simulink model "ackerman_ROS_neural_controller"  (R2023b)
settings: Solver=FixedStepDiscrete  StartTime=0.0  StopTime=20  FixedStep=0.1  RelTol=1e-3
undefined symbols (not defined in the file or in its folder): Angular, Linear
libraries: neural x61, robotlib x15, robotcorelib x1
(part 2 of 3)

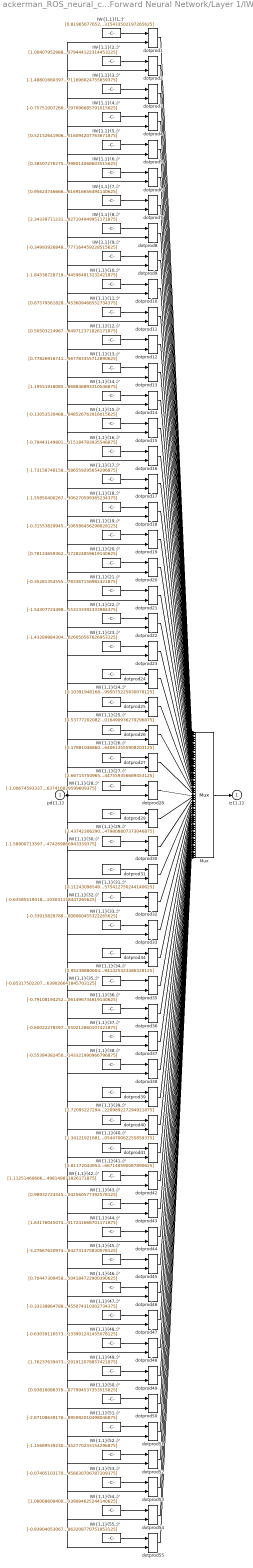
== system ackerman_ROS_neural_controller/Controlador/Feed-Forward Neural Network/Layer 1/IW{1,1} ==
  "pd{1,1}" : Inport  PortDimensions=7
      mask Display: e = 0.06;c1 = [120 230 180]/255;c2 = ([120 230 180]+0)/(256+128);c3 = ([120 230 180]+128)/(256+128);patch([0 1 1 0],[0 0 1 1],c1);patch([0 1 1 1-e 1-e 0+e],[0 0 1 1-e 0+e 0+e],c2);patch([0 0 1 1-e 0+e 0+e],[0 1 1 1-e 1-e 0+e],c3);plot([0 1 1 0 0],[0 0 1 1 0]);
  "IW{1,1}(1,:)'" : Constant  Value=[0.8196567765200553079552037161192856729030609130859375;-1.926081750277442328211918720626272261142730712890625;0.00937690139589171522960242555200238712131977081298828125;-0.99967118914263497497785238010692410171031951904296875;0.88527747342578033684645788525813259184360504150390625;-0.016050046443263653317412575916023342870175838470458984375;2.516567789495900431262498386786319315433502197265625]
      mask Display: e = 0.06;c1 = [120 150 230]/255;c2 = ([120 150 230]+0)/383;c3 = ([120 150 230]+128)/383;patch([0 1 1 0],[0 0 1 1],c1);patch([0 1 1 1-e 1-e 0+e],[0 0 1 1-e 0+e 0+e],c2);patch([0 0 1 1-e 0+e 0+e],[0 1 1 1-e 1-e 0+e],c3);plot([0 1 1 0 0],[0 0 1 1 0]);disp('Weights');
  "IW{1,1}(10,:)'" : Constant  Value=[-1.8453872871921481735313363969908095896244049072265625;1.7100070055517571088188333305879496037960052490234375;-1.2349725100067565630723720460082404315471649169921875;-0.3362332664637464052503901257296092808246612548828125;-1.5013049550553019262366660768748261034488677978515625;0.8324461871242399002568390642409212887287139892578125;-0.88812634608944385217199624094064347445964813232421875]
      mask Display: e = 0.06;c1 = [120 150 230]/255;c2 = ([120 150 230]+0)/383;c3 = ([120 150 230]+128)/383;patch([0 1 1 0],[0 0 1 1],c1);patch([0 1 1 1-e 1-e 0+e],[0 0 1 1-e 0+e 0+e],c2);patch([0 0 1 1-e 0+e 0+e],[0 1 1 1-e 1-e 0+e],c3);plot([0 1 1 0 0],[0 0 1 1 0]);disp('Weights');
  "IW{1,1}(11,:)'" : Constant  Value=[0.87579561828426777392309077185927890241146087646484375;-2.18084780642070175105118323699571192264556884765625;1.2546608949978901303978773285052739083766937255859375;-0.09026831162019467724721977219815016724169254302978515625;-0.07461867636167125727997273543223855085670948028564453125;-0.00755235780173457715847007420961745083332061767578125;0.464016361247922670685284174396656453609466552734375]
      mask Display: e = 0.06;c1 = [120 150 230]/255;c2 = ([120 150 230]+0)/383;c3 = ([120 150 230]+128)/383;patch([0 1 1 0],[0 0 1 1],c1);patch([0 1 1 1-e 1-e 0+e],[0 0 1 1-e 0+e 0+e],c2);patch([0 0 1 1-e 0+e 0+e],[0 1 1 1-e 1-e 0+e],c3);plot([0 1 1 0 0],[0 0 1 1 0]);disp('Weights');
  "IW{1,1}(12,:)'" : Constant  Value=[0.5050321496787890662716336009907536208629608154296875;0.328844036297810060620605554504436440765857696533203125;1.77708828566390497627480726805515587329864501953125;-1.3961094208468234345588143696659244596958160400390625;0.28492086151952722428148945255088619887828826904296875;1.5220770934261285134425634169019758701324462890625;-0.064043810457246663769836914070765487849712371826171875]
      mask Display: e = 0.06;c1 = [120 150 230]/255;c2 = ([120 150 230]+0)/383;c3 = ([120 150 230]+128)/383;patch([0 1 1 0],[0 0 1 1],c1);patch([0 1 1 1-e 1-e 0+e],[0 0 1 1-e 0+e 0+e],c2);patch([0 0 1 1-e 0+e 0+e],[0 1 1 1-e 1-e 0+e],c3);plot([0 1 1 0 0],[0 0 1 1 0]);disp('Weights');
  "IW{1,1}(13,:)'" : Constant  Value=[0.77826916741648866082670110699837096035480499267578125;-0.6526054454813519090095041974564082920551300048828125;1.551566772193030185889028871315531432628631591796875;1.1956969864732924779815448346198536455631256103515625;-1.4944987700257410523363432730548083782196044921875;1.1012912516788346817264709898154251277446746826171875;-0.1254181577627761223769908838221454061567783355712890625]
      mask Display: e = 0.06;c1 = [120 150 230]/255;c2 = ([120 150 230]+0)/383;c3 = ([120 150 230]+128)/383;patch([0 1 1 0],[0 0 1 1],c1);patch([0 1 1 1-e 1-e 0+e],[0 0 1 1-e 0+e 0+e],c2);patch([0 0 1 1-e 0+e 0+e],[0 1 1 1-e 1-e 0+e],c3);plot([0 1 1 0 0],[0 0 1 1 0]);disp('Weights');
  "IW{1,1}(14,:)'" : Constant  Value=[1.195519180856158936165911654825322329998016357421875;1.2214638332623959371403543627820909023284912109375;1.6603997501206200215762009975151158869266510009765625;2.570219412985425666562377955415286123752593994140625;-0.81621421998230847538735588386771269142627716064453125;0.106969592196890561641708927709260024130344390869140625;-0.2002481022235455820901250945098581723868846893310546875]
      mask Display: e = 0.06;c1 = [120 150 230]/255;c2 = ([120 150 230]+0)/383;c3 = ([120 150 230]+128)/383;patch([0 1 1 0],[0 0 1 1],c1);patch([0 1 1 1-e 1-e 0+e],[0 0 1 1-e 0+e 0+e],c2);patch([0 0 1 1-e 0+e 0+e],[0 1 1 1-e 1-e 0+e],c3);plot([0 1 1 0 0],[0 0 1 1 0]);disp('Weights');
  "IW{1,1}(15,:)'" : Constant  Value=[-0.1305353046822148310734945653166505508124828338623046875;0.42887859104116843322884733424871228635311126708984375;-0.1528195850874631833704597738687880337238311767578125;-0.44812624061969741351418861086131073534488677978515625;2.323367873082375911764074771781452000141143798828125;0.09038873200569443044916084772921749390661716461181640625;1.265699700169220509593515089363791048526763916015625]
      mask Display: e = 0.06;c1 = [120 150 230]/255;c2 = ([120 150 230]+0)/383;c3 = ([120 150 230]+128)/383;patch([0 1 1 0],[0 0 1 1],c1);patch([0 1 1 1-e 1-e 0+e],[0 0 1 1-e 0+e 0+e],c2);patch([0 0 1 1-e 0+e 0+e],[0 1 1 1-e 1-e 0+e],c3);plot([0 1 1 0 0],[0 0 1 1 0]);disp('Weights');
  "IW{1,1}(16,:)'" : Constant  Value=[-0.79443149801045287450307341714506037533283233642578125;-1.2581818433612481644701119876117445528507232666015625;0.403920568372703014947688870961428619921207427978515625;-0.9387576041271177285096882769721560180187225341796875;-1.0760361386877399514361286492203362286090850830078125;0.02723946620754004455111640936593175865709781646728515625;2.420834616643684267245362207177095115184783935546875]
      mask Display: e = 0.06;c1 = [120 150 230]/255;c2 = ([120 150 230]+0)/383;c3 = ([120 150 230]+128)/383;patch([0 1 1 0],[0 0 1 1],c1);patch([0 1 1 1-e 1-e 0+e],[0 0 1 1-e 0+e 0+e],c2);patch([0 0 1 1-e 0+e 0+e],[0 1 1 1-e 1-e 0+e],c3);plot([0 1 1 0 0],[0 0 1 1 0]);disp('Weights');
  "IW{1,1}(17,:)'" : Constant  Value=[-1.731587481587970156482469974434934556484222412109375;-1.2350643156762668439796470920555293560028076171875;-0.50287132855106786433196930374833755195140838623046875;-0.52530204840375471775359983439557254314422607421875;1.43947154865100213072537371772341430187225341796875;0.04561385884697267967258227372440160252153873443603515625;0.50957825059342443108079123703646473586559295654296875]
      mask Display: e = 0.06;c1 = [120 150 230]/255;c2 = ([120 150 230]+0)/383;c3 = ([120 150 230]+128)/383;patch([0 1 1 0],[0 0 1 1],c1);patch([0 1 1 1-e 1-e 0+e],[0 0 1 1-e 0+e 0+e],c2);patch([0 0 1 1-e 0+e 0+e],[0 1 1 1-e 1-e 0+e],c3);plot([0 1 1 0 0],[0 0 1 1 0]);disp('Weights');
  "IW{1,1}(18,:)'" : Constant  Value=[-1.5585040026759988673887846744037233293056488037109375;0.109992370714509901663546997951925732195377349853515625;0.82737968051371080235867339069955050945281982421875;1.900815407616306629279279150068759918212890625;0.1491678806411325941549961271448410116136074066162109375;-1.205691924855796681725905727944336831569671630859375;0.060510711771919911683426107629202306270599365234375]
      mask Display: e = 0.06;c1 = [120 150 230]/255;c2 = ([120 150 230]+0)/383;c3 = ([120 150 230]+128)/383;patch([0 1 1 0],[0 0 1 1],c1);patch([0 1 1 1-e 1-e 0+e],[0 0 1 1-e 0+e 0+e],c2);patch([0 0 1 1-e 0+e 0+e],[0 1 1 1-e 1-e 0+e],c3);plot([0 1 1 0 0],[0 0 1 1 0]);disp('Weights');
  "IW{1,1}(19,:)'" : Constant  Value=[-0.315538299455872917054222170918365009129047393798828125;0.259542684982053406539392881313688121736049652099609375;-1.2126404532456895868364199486677534878253936767578125;-5.8374282487121842422084228019230067729949951171875;2.580560676999312352819515581359155476093292236328125;0.54278960426659172977537082260823808610439300537109375;-0.8672580816556649807580470223911106586456298828125]
      mask Display: e = 0.06;c1 = [120 150 230]/255;c2 = ([120 150 230]+0)/383;c3 = ([120 150 230]+128)/383;patch([0 1 1 0],[0 0 1 1],c1);patch([0 1 1 1-e 1-e 0+e],[0 0 1 1-e 0+e 0+e],c2);patch([0 0 1 1-e 0+e 0+e],[0 1 1 1-e 1-e 0+e],c3);plot([0 1 1 0 0],[0 0 1 1 0]);disp('Weights');
  "IW{1,1}(2,:)'" : Constant  Value=[1.00407952988688276008133470895700156688690185546875;1.752935551171999950526014799834229052066802978515625;-1.414218430030616868720017009763978421688079833984375;-0.25046873033662586660597071386291645467281341552734375;-1.9154355127652473722577042281045578420162200927734375;0.1438730267330297907246716704321443103253841400146484375;-0.310184078325510814710952445238945074379444122314453125]
      mask Display: e = 0.06;c1 = [120 150 230]/255;c2 = ([120 150 230]+0)/383;c3 = ([120 150 230]+128)/383;patch([0 1 1 0],[0 0 1 1],c1);patch([0 1 1 1-e 1-e 0+e],[0 0 1 1-e 0+e 0+e],c2);patch([0 0 1 1-e 0+e 0+e],[0 1 1 1-e 1-e 0+e],c3);plot([0 1 1 0 0],[0 0 1 1 0]);disp('Weights');
  "IW{1,1}(20,:)'" : Constant  Value=[0.78124659362565151976554034263244830071926116943359375;0.289651182914616500685411892845877446234226226806640625;-1.350122749788877474230730513227172195911407470703125;-1.5462269165205555498943112979759462177753448486328125;0.32235172181962690185486053451313637197017669677734375;-0.5104310959630049548962915650918148458003997802734375;1.810732280847093367270872477092780172824859619140625]
      mask Display: e = 0.06;c1 = [120 150 230]/255;c2 = ([120 150 230]+0)/383;c3 = ([120 150 230]+128)/383;patch([0 1 1 0],[0 0 1 1],c1);patch([0 1 1 1-e 1-e 0+e],[0 0 1 1-e 0+e 0+e],c2);patch([0 0 1 1-e 0+e 0+e],[0 1 1 1-e 1-e 0+e],c3);plot([0 1 1 0 0],[0 0 1 1 0]);disp('Weights');
  "IW{1,1}(21,:)'" : Constant  Value=[-0.35281354555303534592525238622329197824001312255859375;0.1032751127231832100061836854365537874400615692138671875;0.169498037490068476085269821851397864520549774169921875;-1.163129210222102916105768599663861095905303955078125;-1.516689324515800851855829023406840860843658447265625;-1.50230615007458201404233477660454809665679931640625;0.9213137951345735654484769838745705783367156982421875]
      mask Display: e = 0.06;c1 = [120 150 230]/255;c2 = ([120 150 230]+0)/383;c3 = ([120 150 230]+128)/383;patch([0 1 1 0],[0 0 1 1],c1);patch([0 1 1 1-e 1-e 0+e],[0 0 1 1-e 0+e 0+e],c2);patch([0 0 1 1-e 0+e 0+e],[0 1 1 1-e 1-e 0+e],c3);plot([0 1 1 0 0],[0 0 1 1 0]);disp('Weights');
  "IW{1,1}(22,:)'" : Constant  Value=[-1.543077244984001783478788638603873550891876220703125;1.840093239849561967957924935035407543182373046875;-1.5256171026490890074711614943225868046283721923828125;-0.51244468639139062471343777360743843019008636474609375;0.637896693551966986746037946431897580623626708984375;0.8300709977513041071262023251620121300220489501953125;-1.3458241602968799011108558261184953153133392333984375]
      mask Display: e = 0.06;c1 = [120 150 230]/255;c2 = ([120 150 230]+0)/383;c3 = ([120 150 230]+128)/383;patch([0 1 1 0],[0 0 1 1],c1);patch([0 1 1 1-e 1-e 0+e],[0 0 1 1-e 0+e 0+e],c2);patch([0 0 1 1-e 0+e 0+e],[0 1 1 1-e 1-e 0+e],c3);plot([0 1 1 0 0],[0 0 1 1 0]);disp('Weights');
  "IW{1,1}(23,:)'" : Constant  Value=[-1.43289884304300851880498157697729766368865966796875;1.9791366659345455136786995353759266436100006103515625;0.481076891871465461836265831152559258043766021728515625;-1.2587924341996383770236889176885597407817840576171875;0.2231337452412995581152443946848507039248943328857421875;1.2838954097952697264162225110339932143688201904296875;0.97161406138600459048149105001357384026050567626953125]
      mask Display: e = 0.06;c1 = [120 150 230]/255;c2 = ([120 150 230]+0)/383;c3 = ([120 150 230]+128)/383;patch([0 1 1 0],[0 0 1 1],c1);patch([0 1 1 1-e 1-e 0+e],[0 0 1 1-e 0+e 0+e],c2);patch([0 0 1 1-e 0+e 0+e],[0 1 1 1-e 1-e 0+e],c3);plot([0 1 1 0 0],[0 0 1 1 0]);disp('Weights');
  "IW{1,1}(24,:)'" : Constant  Value=[0.1039194816821370215276232329415506683290004730224609375;-2.24536042172727778876151205622591078281402587890625;0.94414930025091425846994752646423876285552978515625;-0.472618055494270716820892630494199693202972412109375;0.7174481316047778278743862756527960300445556640625;2.271186922768583027476552160806022584438323974609375;2.795885435963406440151857168530113995075225830078125]
      mask Display: e = 0.06;c1 = [120 150 230]/255;c2 = ([120 150 230]+0)/383;c3 = ([120 150 230]+128)/383;patch([0 1 1 0],[0 0 1 1],c1);patch([0 1 1 1-e 1-e 0+e],[0 0 1 1-e 0+e 0+e],c2);patch([0 0 1 1-e 0+e 0+e],[0 1 1 1-e 1-e 0+e],c3);plot([0 1 1 0 0],[0 0 1 1 0]);disp('Weights');
  "IW{1,1}(25,:)'" : Constant  Value=[0.53777202082343311673184871324338018894195556640625;0.52823704471663857074048564754775725305080413818359375;-0.59883371214820979577808657268178649246692657470703125;0.12258232964106541285076446001767180860042572021484375;0.5166091212520906861271896559628657996654510498046875;-0.13458293841771162835385666767251677811145782470703125;0.8974266232529461984057661538827233016490936279296875]
      mask Display: e = 0.06;c1 = [120 150 230]/255;c2 = ([120 150 230]+0)/383;c3 = ([120 150 230]+128)/383;patch([0 1 1 0],[0 0 1 1],c1);patch([0 1 1 1-e 1-e 0+e],[0 0 1 1-e 0+e 0+e],c2);patch([0 0 1 1-e 0+e 0+e],[0 1 1 1-e 1-e 0+e],c3);plot([0 1 1 0 0],[0 0 1 1 0]);disp('Weights');
  "IW{1,1}(26,:)'" : Constant  Value=[0.1788104686056406766869741886694100685417652130126953125;0.330006955410862834465746118439710699021816253662109375;-1.1674892308520219419420982376323081552982330322265625;-2.918953004432601527895485560293309390544891357421875;1.1324442299923582755383222320233471691608428955078125;0.7442867829941091084577919900766573846340179443359375;-0.361699594847931404917318332081777043640613555908203125]
      mask Display: e = 0.06;c1 = [120 150 230]/255;c2 = ([120 150 230]+0)/383;c3 = ([120 150 230]+128)/383;patch([0 1 1 0],[0 0 1 1],c1);patch([0 1 1 1-e 1-e 0+e],[0 0 1 1-e 0+e 0+e],c2);patch([0 0 1 1-e 0+e 0+e],[0 1 1 1-e 1-e 0+e],c3);plot([0 1 1 0 0],[0 0 1 1 0]);disp('Weights');
  "IW{1,1}(27,:)'" : Constant  Value=[2.66715750965894660140520500135608017444610595703125;-2.27722146233000888315700649400241672992706298828125;0.71597217798577694747308441947097890079021453857421875;-1.6139328980116334211203366066911257803440093994140625;1.9382503882814037243775828756042756140232086181640625;-0.2017845621484758711350337989642866887152194976806640625;0.08781462402644509002147543696992215700447559356689453125]
      mask Display: e = 0.06;c1 = [120 150 230]/255;c2 = ([120 150 230]+0)/383;c3 = ([120 150 230]+128)/383;patch([0 1 1 0],[0 0 1 1],c1);patch([0 1 1 1-e 1-e 0+e],[0 0 1 1-e 0+e 0+e],c2);patch([0 0 1 1-e 0+e 0+e],[0 1 1 1-e 1-e 0+e],c3);plot([0 1 1 0 0],[0 0 1 1 0]);disp('Weights');
  "IW{1,1}(28,:)'" : Constant  Value=[-1.006745933372045431752894728560931980609893798828125;-2.0608963324433648978128985618241131305694580078125;0.043165708065044106067631446421728469431400299072265625;0.719486909065246482697375540737994015216827392578125;-0.1733343365394100776821773024494177661836147308349609375;-0.2415300122648019465199098476659855805337429046630859375;-1.1204520286378620852474341518245637416839599609375]
      mask Display: e = 0.06;c1 = [120 150 230]/255;c2 = ([120 150 230]+0)/383;c3 = ([120 150 230]+128)/383;patch([0 1 1 0],[0 0 1 1],c1);patch([0 1 1 1-e 1-e 0+e],[0 0 1 1-e 0+e 0+e],c2);patch([0 0 1 1-e 0+e 0+e],[0 1 1 1-e 1-e 0+e],c3);plot([0 1 1 0 0],[0 0 1 1 0]);disp('Weights');
  "IW{1,1}(29,:)'" : Constant  Value=[2.437423062906741488831130482139997184276580810546875;-2.356093352610267199764848555787466466426849365234375;-1.750998763544374892120458753197453916072845458984375;0.1934240615399113460970426103813224472105503082275390625;-0.11899669455935434070337208822820684872567653656005859375;1.12619821571909550783630038495175540447235107421875;3.56357954247615094089951526257209479808807373046875]
      mask Display: e = 0.06;c1 = [120 150 230]/255;c2 = ([120 150 230]+0)/383;c3 = ([120 150 230]+128)/383;patch([0 1 1 0],[0 0 1 1],c1);patch([0 1 1 1-e 1-e 0+e],[0 0 1 1-e 0+e 0+e],c2);patch([0 0 1 1-e 0+e 0+e],[0 1 1 1-e 1-e 0+e],c3);plot([0 1 1 0 0],[0 0 1 1 0]);disp('Weights');
  "IW{1,1}(3,:)'" : Constant  Value=[-1.4880166039728168758671245086588896811008453369140625;0.245406596910593799432120931669487617909908294677734375;-0.651966682995968493941063570673577487468719482421875;-0.2076135471464277681974408551468513906002044677734375;-0.9089205659120456193278414502856321632862091064453125;1.1562892851109205505366617217077873647212982177734375;-0.6555946798450447143835617680451832711696624755859375]
      mask Display: e = 0.06;c1 = [120 150 230]/255;c2 = ([120 150 230]+0)/383;c3 = ([120 150 230]+128)/383;patch([0 1 1 0],[0 0 1 1],c1);patch([0 1 1 1-e 1-e 0+e],[0 0 1 1-e 0+e 0+e],c2);patch([0 0 1 1-e 0+e 0+e],[0 1 1 1-e 1-e 0+e],c3);plot([0 1 1 0 0],[0 0 1 1 0]);disp('Weights');
  "IW{1,1}(30,:)'" : Constant  Value=[-1.589007135976476359218167999642901122570037841796875;-1.31141949337409879916549471090547740459442138671875;-1.0226840662479588228706006702850572764873504638671875;1.7847567115081093280792856603511609137058258056640625;-0.9266439972251323542451473258552141487598419189453125;-0.00035821150614343856555255030116313719190657138824462890625;1.7299014906363507915187938124290667474269866943359375]
      mask Display: e = 0.06;c1 = [120 150 230]/255;c2 = ([120 150 230]+0)/383;c3 = ([120 150 230]+128)/383;patch([0 1 1 0],[0 0 1 1],c1);patch([0 1 1 1-e 1-e 0+e],[0 0 1 1-e 0+e 0+e],c2);patch([0 0 1 1-e 0+e 0+e],[0 1 1 1-e 1-e 0+e],c3);plot([0 1 1 0 0],[0 0 1 1 0]);disp('Weights');
  "IW{1,1}(31,:)'" : Constant  Value=[0.1124309654881923414837530117438291199505329132080078125;0.029087691018045168378503007033941685222089290618896484375;-1.055713623776400655884799562045373022556304931640625;0.93835294125979340496002123472862876951694488525390625;1.4852531373823329996497477623051963746547698974609375;-0.388212588822750614969692151134950108826160430908203125;-1.2185456909971110750490197460749186575412750244140625]
      mask Display: e = 0.06;c1 = [120 150 230]/255;c2 = ([120 150 230]+0)/383;c3 = ([120 150 230]+128)/383;patch([0 1 1 0],[0 0 1 1],c1);patch([0 1 1 1-e 1-e 0+e],[0 0 1 1-e 0+e 0+e],c2);patch([0 0 1 1-e 0+e 0+e],[0 1 1 1-e 1-e 0+e],c3);plot([0 1 1 0 0],[0 0 1 1 0]);disp('Weights');
  "IW{1,1}(32,:)'" : Constant  Value=[-0.63585519418358427135018473563832230865955352783203125;-1.5254086535969004767565593283507041633129119873046875;0.3019815538911905239416455515311099588871002197265625;0.5804630405005115623140454772510565817356109619140625;-1.937194029410040929661818154272623360157012939453125;-0.470855409083529574676418860690318979322910308837890625;-1.2814806828813607442185684703872539103031158447265625]
      mask Display: e = 0.06;c1 = [120 150 230]/255;c2 = ([120 150 230]+0)/383;c3 = ([120 150 230]+128)/383;patch([0 1 1 0],[0 0 1 1],c1);patch([0 1 1 1-e 1-e 0+e],[0 0 1 1-e 0+e 0+e],c2);patch([0 0 1 1-e 0+e 0+e],[0 1 1 1-e 1-e 0+e],c3);plot([0 1 1 0 0],[0 0 1 1 0]);disp('Weights');
  "IW{1,1}(33,:)'" : Constant  Value=[-0.33915828788690050021870092678000219166278839111328125;0.1789708238793852601578038274965365417301654815673828125;0.970370936337600742405129494727589190006256103515625;3.0714089604893803908680638414807617664337158203125;-1.5686418166151068209757113436353392899036407470703125;0.658094509689622686465781953302212059497833251953125;-1.5427494403949657542085560635314323008060455322265625]
      mask Display: e = 0.06;c1 = [120 150 230]/255;c2 = ([120 150 230]+0)/383;c3 = ([120 150 230]+128)/383;patch([0 1 1 0],[0 0 1 1],c1);patch([0 1 1 1-e 1-e 0+e],[0 0 1 1-e 0+e 0+e],c2);patch([0 0 1 1-e 0+e 0+e],[0 1 1 1-e 1-e 0+e],c3);plot([0 1 1 0 0],[0 0 1 1 0]);disp('Weights');
  "IW{1,1}(34,:)'" : Constant  Value=[0.95238880604200115698176887235604226589202880859375;-0.24816195974321664241557527930126525461673736572265625;0.322253882548174719335776217121747322380542755126953125;-1.99655520246268025630342890508472919464111328125;-1.0472174516072503269725757490959949791431427001953125;0.163076430626699797610257292035385034978389739990234375;0.66808023651050973956699863265384919941425323486328125]
      mask Display: e = 0.06;c1 = [120 150 230]/255;c2 = ([120 150 230]+0)/383;c3 = ([120 150 230]+128)/383;patch([0 1 1 0],[0 0 1 1],c1);patch([0 1 1 1-e 1-e 0+e],[0 0 1 1-e 0+e 0+e],c2);patch([0 0 1 1-e 0+e 0+e],[0 1 1 1-e 1-e 0+e],c3);plot([0 1 1 0 0],[0 0 1 1 0]);disp('Weights');
  "IW{1,1}(35,:)'" : Constant  Value=[-0.85317502207466178187900140983401797711849212646484375;-1.4926232868599556002919825914432294666767120361328125;-1.661914641538658532482486407388933002948760986328125;1.0289793115468095496822797940694727003574371337890625;-1.1862452665797944550973852528841234743595123291015625;0.75256474756981639462338762314175255596637725830078125;1.4295861162861112081401415707659907639026641845703125]
      mask Display: e = 0.06;c1 = [120 150 230]/255;c2 = ([120 150 230]+0)/383;c3 = ([120 150 230]+128)/383;patch([0 1 1 0],[0 0 1 1],c1);patch([0 1 1 1-e 1-e 0+e],[0 0 1 1-e 0+e 0+e],c2);patch([0 0 1 1-e 0+e 0+e],[0 1 1 1-e 1-e 0+e],c3);plot([0 1 1 0 0],[0 0 1 1 0]);disp('Weights');
  "IW{1,1}(36,:)'" : Constant  Value=[-0.7910819425205526389532906250678934156894683837890625;-1.22567617800795591875839818385429680347442626953125;1.3861154071558396960739401038154028356075286865234375;1.407270113114253984321067036944441497325897216796875;-0.7349364898058803330371802076115272939205169677734375;0.1550965372921388196747471965863951481878757476806640625;0.90868774255624418234589256826438941061496734619140625]
      mask Display: e = 0.06;c1 = [120 150 230]/255;c2 = ([120 150 230]+0)/383;c3 = ([120 150 230]+128)/383;patch([0 1 1 0],[0 0 1 1],c1);patch([0 1 1 1-e 1-e 0+e],[0 0 1 1-e 0+e 0+e],c2);patch([0 0 1 1-e 0+e 0+e],[0 1 1 1-e 1-e 0+e],c3);plot([0 1 1 0 0],[0 0 1 1 0]);disp('Weights');
  "IW{1,1}(37,:)'" : Constant  Value=[-0.60022278597785827525257218439946882426738739013671875;-1.37806659108217655074213325860910117626190185546875;-0.303251482179367204405906477404641918838024139404296875;1.37025136930491253650643557193689048290252685546875;-1.4462899506258259929580844982410781085491180419921875;-0.88906156361151256195540781845920719206333160400390625;2.554269484025119663073155606980435550212860107421875]
      mask Display: e = 0.06;c1 = [120 150 230]/255;c2 = ([120 150 230]+0)/383;c3 = ([120 150 230]+128)/383;patch([0 1 1 0],[0 0 1 1],c1);patch([0 1 1 1-e 1-e 0+e],[0 0 1 1-e 0+e 0+e],c2);patch([0 0 1 1-e 0+e 0+e],[0 1 1 1-e 1-e 0+e],c3);plot([0 1 1 0 0],[0 0 1 1 0]);disp('Weights');
  "IW{1,1}(38,:)'" : Constant  Value=[-0.5539438245094190360617858459590934216976165771484375;-0.7584753336702918513623217222630046308040618896484375;1.1244270998492973401283734347089193761348724365234375;0.92108337779718507665194238143158145248889923095703125;1.2173327787359589091664702209527604281902313232421875;-1.1346602437829156340143299530609510838985443115234375;1.36923191299962621059194134431891143321990966796875]
      mask Display: e = 0.06;c1 = [120 150 230]/255;c2 = ([120 150 230]+0)/383;c3 = ([120 150 230]+128)/383;patch([0 1 1 0],[0 0 1 1],c1);patch([0 1 1 1-e 1-e 0+e],[0 0 1 1-e 0+e 0+e],c2);patch([0 0 1 1-e 0+e 0+e],[0 1 1 1-e 1-e 0+e],c3);plot([0 1 1 0 0],[0 0 1 1 0]);disp('Weights');
  "IW{1,1}(39,:)'" : Constant  Value=[2.7209522729420285713786142878234386444091796875;-1.0945334463846523309626945774652995169162750244140625;0.157552272685574756838633447841857559978961944580078125;-0.394241827597444249864366838664864189922809600830078125;1.660163967521395722570787256699986755847930908203125;1.012816418846511634654916633735410869121551513671875;-0.341829665721035957925977299964870326220989227294921875]
      mask Display: e = 0.06;c1 = [120 150 230]/255;c2 = ([120 150 230]+0)/383;c3 = ([120 150 230]+128)/383;patch([0 1 1 0],[0 0 1 1],c1);patch([0 1 1 1-e 1-e 0+e],[0 0 1 1-e 0+e 0+e],c2);patch([0 0 1 1-e 0+e 0+e],[0 1 1 1-e 1-e 0+e],c3);plot([0 1 1 0 0],[0 0 1 1 0]);disp('Weights');
  "IW{1,1}(4,:)'" : Constant  Value=[-0.7575100726613366308725971975945867598056793212890625;0.6413715582514225577170918768388219177722930908203125;-0.327350184006029387706604438790236599743366241455078125;0.16818639155169534671330211494932882487773895263671875;1.5231808779497211236986231597256846725940704345703125;1.4489465731582369389940367909730412065982818603515625;1.1133057349200383701059990926296450197696685791015625]
      mask Display: e = 0.06;c1 = [120 150 230]/255;c2 = ([120 150 230]+0)/383;c3 = ([120 150 230]+128)/383;patch([0 1 1 0],[0 0 1 1],c1);patch([0 1 1 1-e 1-e 0+e],[0 0 1 1-e 0+e 0+e],c2);patch([0 0 1 1-e 0+e 0+e],[0 1 1 1-e 1-e 0+e],c3);plot([0 1 1 0 0],[0 0 1 1 0]);disp('Weights');
  "IW{1,1}(40,:)'" : Constant  Value=[1.341219216816540438230731524527072906494140625;-1.280045153834659998892675503157079219818115234375;-1.1552678395764088836727978559792973101139068603515625;-1.0172734670797767275729484026669524610042572021484375;-1.896706345967122953055650214082561433315277099609375;-1.9325992429389244886550613955478183925151824951171875;-0.2310712980003092054115398923386237584054470062255859375]
      mask Display: e = 0.06;c1 = [120 150 230]/255;c2 = ([120 150 230]+0)/383;c3 = ([120 150 230]+128)/383;patch([0 1 1 0],[0 0 1 1],c1);patch([0 1 1 1-e 1-e 0+e],[0 0 1 1-e 0+e 0+e],c2);patch([0 0 1 1-e 0+e 0+e],[0 1 1 1-e 1-e 0+e],c3);plot([0 1 1 0 0],[0 0 1 1 0]);disp('Weights');
  "IW{1,1}(41,:)'" : Constant  Value=[0.811720449545865196938621011213399469852447509765625;-1.6561488284375922575009099091403186321258544921875;-1.7328728550059857571596921843593008816242218017578125;-0.21385112741317102713622944065718911588191986083984375;1.500831725264960336829744846909306943416595458984375;1.9648776647549202056808326233294792473316192626953125;2.765549270180410079689181657158769667148590087890625]
      mask Display: e = 0.06;c1 = [120 150 230]/255;c2 = ([120 150 230]+0)/383;c3 = ([120 150 230]+128)/383;patch([0 1 1 0],[0 0 1 1],c1);patch([0 1 1 1-e 1-e 0+e],[0 0 1 1-e 0+e 0+e],c2);patch([0 0 1 1-e 0+e 0+e],[0 1 1 1-e 1-e 0+e],c3);plot([0 1 1 0 0],[0 0 1 1 0]);disp('Weights');
  "IW{1,1}(42,:)'" : Constant  Value=[1.1125146066644464593053953649359755218029022216796875;0.97245447228481374235542489259387366473674774169921875;-0.09357073027608908688534938846714794635772705078125;-0.52143578599558271235991924186237156391143798828125;1.6900453169367322114879925720742903649806976318359375;0.89353993684356536331137021988979540765285491943359375;0.15465639019748678162358146437327377498149871826171875]
      mask Display: e = 0.06;c1 = [120 150 230]/255;c2 = ([120 150 230]+0)/383;c3 = ([120 150 230]+128)/383;patch([0 1 1 0],[0 0 1 1],c1);patch([0 1 1 1-e 1-e 0+e],[0 0 1 1-e 0+e 0+e],c2);patch([0 0 1 1-e 0+e 0+e],[0 1 1 1-e 1-e 0+e],c3);plot([0 1 1 0 0],[0 0 1 1 0]);disp('Weights');
  "IW{1,1}(43,:)'" : Constant  Value=[0.98932724545203309940433200608822517096996307373046875;-1.159039771877323321547237355844117701053619384765625;-1.2936909148573523253844541613943874835968017578125;-5.8052772640651522095822656410746276378631591796875;1.6865724615037958056262823447468690574169158935546875;0.028487382000130227754919332028293865732848644256591796875;-0.5414572881857886432754867200856097042560577392578125]
      mask Display: e = 0.06;c1 = [120 150 230]/255;c2 = ([120 150 230]+0)/383;c3 = ([120 150 230]+128)/383;patch([0 1 1 0],[0 0 1 1],c1);patch([0 1 1 1-e 1-e 0+e],[0 0 1 1-e 0+e 0+e],c2);patch([0 0 1 1-e 0+e 0+e],[0 1 1 1-e 1-e 0+e],c3);plot([0 1 1 0 0],[0 0 1 1 0]);disp('Weights');
  "IW{1,1}(44,:)'" : Constant  Value=[1.631760450745726842569638392888009548187255859375;-0.3383095368522173185255041971686296164989471435546875;0.1577241905463775684115290687259403057396411895751953125;1.5203158379761558816056776777259074151515960693359375;0.1856030836735037825580008075121440924704074859619140625;0.96868420701784441195769659316283650696277618408203125;-0.2941332291259513009862303078989498317241668701171875]
      mask Display: e = 0.06;c1 = [120 150 230]/255;c2 = ([120 150 230]+0)/383;c3 = ([120 150 230]+128)/383;patch([0 1 1 0],[0 0 1 1],c1);patch([0 1 1 1-e 1-e 0+e],[0 0 1 1-e 0+e 0+e],c2);patch([0 0 1 1-e 0+e 0+e],[0 1 1 1-e 1-e 0+e],c3);plot([0 1 1 0 0],[0 0 1 1 0]);disp('Weights');
  "IW{1,1}(45,:)'" : Constant  Value=[-3.2766762097488193461458649835549294948577880859375;3.5024319221616888597736760857515037059783935546875;1.1214186183344254654770111301331780850887298583984375;1.31610510688262305478701819083653390407562255859375;-2.069485394238769426777935223071835935115814208984375;-1.1759152851278626972231222680420614778995513916015625;-2.083225199012155304245652587269432842731475830078125]
      mask Display: e = 0.06;c1 = [120 150 230]/255;c2 = ([120 150 230]+0)/383;c3 = ([120 150 230]+128)/383;patch([0 1 1 0],[0 0 1 1],c1);patch([0 1 1 1-e 1-e 0+e],[0 0 1 1-e 0+e 0+e],c2);patch([0 0 1 1-e 0+e 0+e],[0 1 1 1-e 1-e 0+e],c3);plot([0 1 1 0 0],[0 0 1 1 0]);disp('Weights');
  "IW{1,1}(46,:)'" : Constant  Value=[0.70447309458965445827516305143944919109344482421875;1.116325241744835938817459464189596474170684814453125;1.1719149962083028615467128474847413599491119384765625;-0.2078362875385108277104251328637474216520786285400390625;-1.724921433949320626055623506545089185237884521484375;0.5326757694421517808081034672795794904232025146484375;-0.1411904022038809325412245243569486774504184722900390625]
      mask Display: e = 0.06;c1 = [120 150 230]/255;c2 = ([120 150 230]+0)/383;c3 = ([120 150 230]+128)/383;patch([0 1 1 0],[0 0 1 1],c1);patch([0 1 1 1-e 1-e 0+e],[0 0 1 1-e 0+e 0+e],c2);patch([0 0 1 1-e 0+e 0+e],[0 1 1 1-e 1-e 0+e],c3);plot([0 1 1 0 0],[0 0 1 1 0]);disp('Weights');
  "IW{1,1}(47,:)'" : Constant  Value=[-0.3323886478852517978310743274050764739513397216796875;1.362359066339624558139576038229279220104217529296875;0.660898331933821747696811144123785197734832763671875;2.014550133953556088073355567757971584796905517578125;-1.18255180022787786953131217160262167453765869140625;1.073171118143467328565066054579801857471466064453125;0.377789546655022456800310237667872570455074310302734375]
      mask Display: e = 0.06;c1 = [120 150 230]/255;c2 = ([120 150 230]+0)/383;c3 = ([120 150 230]+128)/383;patch([0 1 1 0],[0 0 1 1],c1);patch([0 1 1 1-e 1-e 0+e],[0 0 1 1-e 0+e 0+e],c2);patch([0 0 1 1-e 0+e 0+e],[0 1 1 1-e 1-e 0+e],c3);plot([0 1 1 0 0],[0 0 1 1 0]);disp('Weights');
  "IW{1,1}(48,:)'" : Constant  Value=[-0.630391165733994451869648401043377816677093505859375;-0.0153976369140470491225780591548755182884633541107177734375;0.57130765059060839572424583820975385606288909912109375;-1.6250766129481573063486621322226710617542266845703125;-0.590198279604056796898703396436758339405059814453125;-1.5454180687105976144124497295706532895565032958984375;0.80812970449453580545906561383162625133991241455078125]
      mask Display: e = 0.06;c1 = [120 150 230]/255;c2 = ([120 150 230]+0)/383;c3 = ([120 150 230]+128)/383;patch([0 1 1 0],[0 0 1 1],c1);patch([0 1 1 1-e 1-e 0+e],[0 0 1 1-e 0+e 0+e],c2);patch([0 0 1 1-e 0+e 0+e],[0 1 1 1-e 1-e 0+e],c3);plot([0 1 1 0 0],[0 0 1 1 0]);disp('Weights');
  "IW{1,1}(49,:)'" : Constant  Value=[1.7623763947340425062293434166349470615386962890625;0.1122253077224798223365809235474443994462490081787109375;-1.0793826107514450374225134510197676718235015869140625;1.1913612470027936662830825298442505300045013427734375;-0.3088869039969164287384728595498017966747283935546875;-0.34303903022608162043383117634220980107784271240234375;0.344119634973915899944785223851795308291912078857421875]
      mask Display: e = 0.06;c1 = [120 150 230]/255;c2 = ([120 150 230]+0)/383;c3 = ([120 150 230]+128)/383;patch([0 1 1 0],[0 0 1 1],c1);patch([0 1 1 1-e 1-e 0+e],[0 0 1 1-e 0+e 0+e],c2);patch([0 0 1 1-e 0+e 0+e],[0 1 1 1-e 1-e 0+e],c3);plot([0 1 1 0 0],[0 0 1 1 0]);disp('Weights');
  "IW{1,1}(5,:)'" : Constant  Value=[0.521526419068620850083561890642158687114715576171875;-0.93302138605841833385312611426343210041522979736328125;0.91289092879218280973674382039462216198444366455078125;-0.8899023001811785515968722393154166638851165771484375;-1.4775644486773205077412285390892066061496734619140625;-1.258156522644350072681618257774971425533294677734375;0.271794374927213311377016680125962011516094207763671875]
      mask Display: e = 0.06;c1 = [120 150 230]/255;c2 = ([120 150 230]+0)/383;c3 = ([120 150 230]+128)/383;patch([0 1 1 0],[0 0 1 1],c1);patch([0 1 1 1-e 1-e 0+e],[0 0 1 1-e 0+e 0+e],c2);patch([0 0 1 1-e 0+e 0+e],[0 1 1 1-e 1-e 0+e],c3);plot([0 1 1 0 0],[0 0 1 1 0]);disp('Weights');
  "IW{1,1}(50,:)'" : Constant  Value=[0.938160863796301480732608979451470077037811279296875;1.3162523708538389488609254840412177145481109619140625;-0.117164255967228569943472393788397312164306640625;0.79194042132034947467644769858452491462230682373046875;-1.145429229066855736363095275009982287883758544921875;-1.142466201162294137105845948099158704280853271484375;-0.75608338041751166347381740706623531877994537353515625]
      mask Display: e = 0.06;c1 = [120 150 230]/255;c2 = ([120 150 230]+0)/383;c3 = ([120 150 230]+128)/383;patch([0 1 1 0],[0 0 1 1],c1);patch([0 1 1 1-e 1-e 0+e],[0 0 1 1-e 0+e 0+e],c2);patch([0 0 1 1-e 0+e 0+e],[0 1 1 1-e 1-e 0+e],c3);plot([0 1 1 0 0],[0 0 1 1 0]);disp('Weights');
  "IW{1,1}(51,:)'" : Constant  Value=[-2.87108639176751889721117549925111234188079833984375;0.18010958994591685922159740584902465343475341796875;-0.54250423007459491753223801424610428512096405029296875;0.50347109306742632295339490156038664281368255615234375;0.8724234401445813968933862270205281674861907958984375;1.133381316645864611558636170229874551296234130859375;-0.67648267815359897081606277424725703895092010498046875]
      mask Display: e = 0.06;c1 = [120 150 230]/255;c2 = ([120 150 230]+0)/383;c3 = ([120 150 230]+128)/383;patch([0 1 1 0],[0 0 1 1],c1);patch([0 1 1 1-e 1-e 0+e],[0 0 1 1-e 0+e 0+e],c2);patch([0 0 1 1-e 0+e 0+e],[0 1 1 1-e 1-e 0+e],c3);plot([0 1 1 0 0],[0 0 1 1 0]);disp('Weights');
  "IW{1,1}(52,:)'" : Constant  Value=[-1.156895392305774095120796118862926959991455078125;0.946662633442617806878160990891046822071075439453125;0.6998597378332986895799194826395250856876373291015625;-0.68004780546202614477380166135844774544239044189453125;-1.27249687594937643808634675224311649799346923828125;-0.2213100582333173138582793626483180560171604156494140625;0.44446411624932469219828590212273411452770233154296875]
      mask Display: e = 0.06;c1 = [120 150 230]/255;c2 = ([120 150 230]+0)/383;c3 = ([120 150 230]+128)/383;patch([0 1 1 0],[0 0 1 1],c1);patch([0 1 1 1-e 1-e 0+e],[0 0 1 1-e 0+e 0+e],c2);patch([0 0 1 1-e 0+e 0+e],[0 1 1 1-e 1-e 0+e],c3);plot([0 1 1 0 0],[0 0 1 1 0]);disp('Weights');
  "IW{1,1}(53,:)'" : Constant  Value=[-0.0740510317061175704633768646090175025165081024169921875;-0.63620873768682184579148497505229897797107696533203125;-0.39674733068331657914740162595990113914012908935546875;-1.5890782763189204018772215931676328182220458984375;-0.01085028363347284585671559398178942501544952392578125;1.08307175463415727989513470674864947795867919921875;-0.97423607359150243834022830924368463456630706787109375]
      mask Display: e = 0.06;c1 = [120 150 230]/255;c2 = ([120 150 230]+0)/383;c3 = ([120 150 230]+128)/383;patch([0 1 1 0],[0 0 1 1],c1);patch([0 1 1 1-e 1-e 0+e],[0 0 1 1-e 0+e 0+e],c2);patch([0 0 1 1-e 0+e 0+e],[0 1 1 1-e 1-e 0+e],c3);plot([0 1 1 0 0],[0 0 1 1 0]);disp('Weights');
  "IW{1,1}(54,:)'" : Constant  Value=[1.0806860940013101046730525922612287104129791259765625;1.1716841999886924430285262133111245930194854736328125;0.42171085210198011594684430747292935848236083984375;0.7629892521059102872271751039079390466213226318359375;-1.211875410783021411731397165567614138126373291015625;0.5395915829069364288983479127637110650539398193359375;1.20712999928394371096374015905894339084625244140625]
      mask Display: e = 0.06;c1 = [120 150 230]/255;c2 = ([120 150 230]+0)/383;c3 = ([120 150 230]+128)/383;patch([0 1 1 0],[0 0 1 1],c1);patch([0 1 1 1-e 1-e 0+e],[0 0 1 1-e 0+e 0+e],c2);patch([0 0 1 1-e 0+e 0+e],[0 1 1 1-e 1-e 0+e],c3);plot([0 1 1 0 0],[0 0 1 1 0]);disp('Weights');
  "IW{1,1}(55,:)'" : Constant  Value=[-0.93904053067649562169805221856222487986087799072265625;0.000393862070127380821914220287993657620972953736782073974609375;1.165943672491369653698711772449314594268798828125;1.19108179755135079602723635616712272167205810546875;0.90043892477947828911766237069969065487384796142578125;-0.37966321747893350124769540343550033867359161376953125;0.1115590106219901400663729873485863208770751953125]
      mask Display: e = 0.06;c1 = [120 150 230]/255;c2 = ([120 150 230]+0)/383;c3 = ([120 150 230]+128)/383;patch([0 1 1 0],[0 0 1 1],c1);patch([0 1 1 1-e 1-e 0+e],[0 0 1 1-e 0+e 0+e],c2);patch([0 0 1 1-e 0+e 0+e],[0 1 1 1-e 1-e 0+e],c3);plot([0 1 1 0 0],[0 0 1 1 0]);disp('Weights');
  "IW{1,1}(6,:)'" : Constant  Value=[0.385072762751662744928893289397819899022579193115234375;1.562732408095400149505849185516126453876495361328125;-0.73598543357794221630996389649226330220699310302734375;0.040469623236920881925726689587463624775409698486328125;-1.478663113202756118624847658793441951274871826171875;1.2393778004918341029139128295355476438999176025390625;-1.2603550028624523893228115412057377398014068603515625]
      mask Display: e = 0.06;c1 = [120 150 230]/255;c2 = ([120 150 230]+0)/383;c3 = ([120 150 230]+128)/383;patch([0 1 1 0],[0 0 1 1],c1);patch([0 1 1 1-e 1-e 0+e],[0 0 1 1-e 0+e 0+e],c2);patch([0 0 1 1-e 0+e 0+e],[0 1 1 1-e 1-e 0+e],c3);plot([0 1 1 0 0],[0 0 1 1 0]);disp('Weights');
  "IW{1,1}(7,:)'" : Constant  Value=[0.95624746666433380060112767750979401171207427978515625;-1.50328268878952453491137930541299283504486083984375;-0.07202361237724319575903564327745698392391204833984375;-0.54415099803926059163217132663703523576259613037109375;-3.171317019616967325390533005702309310436248779296875;-0.7575771289964325916344023426063358783721923828125;1.5218329099630596434877816136577166616916656494140625]
      mask Display: e = 0.06;c1 = [120 150 230]/255;c2 = ([120 150 230]+0)/383;c3 = ([120 150 230]+128)/383;patch([0 1 1 0],[0 0 1 1],c1);patch([0 1 1 1-e 1-e 0+e],[0 0 1 1-e 0+e 0+e],c2);patch([0 0 1 1-e 0+e 0+e],[0 1 1 1-e 1-e 0+e],c3);plot([0 1 1 0 0],[0 0 1 1 0]);disp('Weights');
  "IW{1,1}(8,:)'" : Constant  Value=[2.343397112314738794935919941053725779056549072265625;-0.199253204632954261654731453745625913143157958984375;-0.83010742637487766604209582510520704090595245361328125;1.1575597315243950635732517184806056320667266845703125;0.059656626436852024097934332758086384274065494537353515625;-1.93468441146076042258528104866854846477508544921875;0.62022080519887523575306431666831485927104949951171875]
      mask Display: e = 0.06;c1 = [120 150 230]/255;c2 = ([120 150 230]+0)/383;c3 = ([120 150 230]+128)/383;patch([0 1 1 0],[0 0 1 1],c1);patch([0 1 1 1-e 1-e 0+e],[0 0 1 1-e 0+e 0+e],c2);patch([0 0 1 1-e 0+e 0+e],[0 1 1 1-e 1-e 0+e],c3);plot([0 1 1 0 0],[0 0 1 1 0]);disp('Weights');
  "IW{1,1}(9,:)'" : Constant  Value=[-0.349939268487058752210572265539667569100856781005859375;0.455451574156257754655285907574580051004886627197265625;-0.5875488641911295051301067360327579081058502197265625;-1.616888319885245284268648902070708572864532470703125;0.413397466036332927874497045195312239229679107666015625;2.022365526218292242077723130933009088039398193359375;-0.2480196251896357451105501468191505409777164459228515625]
      mask Display: e = 0.06;c1 = [120 150 230]/255;c2 = ([120 150 230]+0)/383;c3 = ([120 150 230]+128)/383;patch([0 1 1 0],[0 0 1 1],c1);patch([0 1 1 1-e 1-e 0+e],[0 0 1 1-e 0+e 0+e],c2);patch([0 0 1 1-e 0+e 0+e],[0 1 1 1-e 1-e 0+e],c3);plot([0 1 1 0 0],[0 0 1 1 0]);disp('Weights');
  Mux : Mux  Inputs=55
      mask Display: e = 0.06;c1 = [120 150 230]/255;c2 = ([120 150 230]+0)/383;c3 = ([120 150 230]+128)/383;patch([0 1 1 0],[0 0 1 1],c1);patch([0 1 1 1-e 1-e 0+e],[0 0 1 1-e 0+e 0+e],c2);patch([0 0 1 1-e 0+e 0+e],[0 1 1 1-e 1-e 0+e],c3);plot([0 1 1 0 0],[0 0 1 1 0]);disp('Mux');
  dotprod{1..55} (55 alike) : neural/Weight Functions/dotprod
  "iz{1,1}" : Outport
      mask Display: e = 0.06;c1 = [120 230 180]/255;c2 = ([120 230 180]+0)/(256+128);c3 = ([120 230 180]+128)/(256+128);patch([0 1 1 0],[0 0 1 1],c1);patch([0 1 1 1-e 1-e 0+e],[0 0 1 1-e 0+e 0+e],c2);patch([0 0 1 1-e 0+e 0+e],[0 1 1 1-e 1-e 0+e],c3);plot([0 1 1 0 0],[0 0 1 1 0]);
  wires:
  "IW{1,1}(1,:)'"/1 -> dotprod1/1
  "pd{1,1}"/1 -> dotprod1/2, dotprod2/2, dotprod3/2, dotprod4/2, dotprod5/2, dotprod6/2, dotprod7/2, dotprod8/2, dotprod9/2, dotprod10/2, dotprod11/2, dotprod12/2, dotprod13/2, dotprod14/2, dotprod15/2, dotprod16/2, dotprod17/2, dotprod18/2, dotprod19/2, dotprod20/2, dotprod21/2, dotprod22/2, dotprod23/2, dotprod24/2, dotprod25/2, dotprod26/2, dotprod27/2, dotprod28/2, dotprod29/2, dotprod30/2, dotprod31/2, dotprod32/2, dotprod33/2, dotprod34/2, dotprod35/2, dotprod36/2, dotprod37/2, dotprod38/2, dotprod39/2, dotprod40/2, dotprod41/2, dotprod42/2, dotprod43/2, dotprod44/2, dotprod45/2, dotprod46/2, dotprod47/2, dotprod48/2, dotprod49/2, dotprod50/2, dotprod51/2, dotprod52/2, dotprod53/2, dotprod54/2, dotprod55/2
  dotprod1/1 -> Mux/1
  "IW{1,1}(2,:)'"/1 -> dotprod2/1
  dotprod2/1 -> Mux/2
  "IW{1,1}(3,:)'"/1 -> dotprod3/1
  dotprod3/1 -> Mux/3
  "IW{1,1}(4,:)'"/1 -> dotprod4/1
  dotprod4/1 -> Mux/4
  "IW{1,1}(5,:)'"/1 -> dotprod5/1
  dotprod5/1 -> Mux/5
  "IW{1,1}(6,:)'"/1 -> dotprod6/1
  dotprod6/1 -> Mux/6
  "IW{1,1}(7,:)'"/1 -> dotprod7/1
  dotprod7/1 -> Mux/7
  "IW{1,1}(8,:)'"/1 -> dotprod8/1
  dotprod8/1 -> Mux/8
  "IW{1,1}(9,:)'"/1 -> dotprod9/1
  dotprod9/1 -> Mux/9
  "IW{1,1}(10,:)'"/1 -> dotprod10/1
  dotprod10/1 -> Mux/10
  "IW{1,1}(11,:)'"/1 -> dotprod11/1
  dotprod11/1 -> Mux/11
  "IW{1,1}(12,:)'"/1 -> dotprod12/1
  dotprod12/1 -> Mux/12
  "IW{1,1}(13,:)'"/1 -> dotprod13/1
  dotprod13/1 -> Mux/13
  "IW{1,1}(14,:)'"/1 -> dotprod14/1
  dotprod14/1 -> Mux/14
  "IW{1,1}(15,:)'"/1 -> dotprod15/1
  dotprod15/1 -> Mux/15
  "IW{1,1}(16,:)'"/1 -> dotprod16/1
  dotprod16/1 -> Mux/16
  "IW{1,1}(17,:)'"/1 -> dotprod17/1
  dotprod17/1 -> Mux/17
  "IW{1,1}(18,:)'"/1 -> dotprod18/1
  dotprod18/1 -> Mux/18
  "IW{1,1}(19,:)'"/1 -> dotprod19/1
  dotprod19/1 -> Mux/19
  "IW{1,1}(20,:)'"/1 -> dotprod20/1
  dotprod20/1 -> Mux/20
  "IW{1,1}(21,:)'"/1 -> dotprod21/1
  dotprod21/1 -> Mux/21
  "IW{1,1}(22,:)'"/1 -> dotprod22/1
  dotprod22/1 -> Mux/22
  "IW{1,1}(23,:)'"/1 -> dotprod23/1
  dotprod23/1 -> Mux/23
  "IW{1,1}(24,:)'"/1 -> dotprod24/1
  dotprod24/1 -> Mux/24
  "IW{1,1}(25,:)'"/1 -> dotprod25/1
  dotprod25/1 -> Mux/25
  "IW{1,1}(26,:)'"/1 -> dotprod26/1
  dotprod26/1 -> Mux/26
  "IW{1,1}(27,:)'"/1 -> dotprod27/1
  dotprod27/1 -> Mux/27
  "IW{1,1}(28,:)'"/1 -> dotprod28/1
  dotprod28/1 -> Mux/28
  "IW{1,1}(29,:)'"/1 -> dotprod29/1
  dotprod29/1 -> Mux/29
  "IW{1,1}(30,:)'"/1 -> dotprod30/1
  dotprod30/1 -> Mux/30
  "IW{1,1}(31,:)'"/1 -> dotprod31/1
  dotprod31/1 -> Mux/31
  "IW{1,1}(32,:)'"/1 -> dotprod32/1
  dotprod32/1 -> Mux/32
  "IW{1,1}(33,:)'"/1 -> dotprod33/1
  dotprod33/1 -> Mux/33
  "IW{1,1}(34,:)'"/1 -> dotprod34/1
  dotprod34/1 -> Mux/34
  "IW{1,1}(35,:)'"/1 -> dotprod35/1
  dotprod35/1 -> Mux/35
  "IW{1,1}(36,:)'"/1 -> dotprod36/1
  dotprod36/1 -> Mux/36
  "IW{1,1}(37,:)'"/1 -> dotprod37/1
  dotprod37/1 -> Mux/37
  "IW{1,1}(38,:)'"/1 -> dotprod38/1
  dotprod38/1 -> Mux/38
  "IW{1,1}(39,:)'"/1 -> dotprod39/1
  dotprod39/1 -> Mux/39
  "IW{1,1}(40,:)'"/1 -> dotprod40/1
  dotprod40/1 -> Mux/40
  "IW{1,1}(41,:)'"/1 -> dotprod41/1
  dotprod41/1 -> Mux/41
  "IW{1,1}(42,:)'"/1 -> dotprod42/1
  dotprod42/1 -> Mux/42
  "IW{1,1}(43,:)'"/1 -> dotprod43/1
  dotprod43/1 -> Mux/43
  "IW{1,1}(44,:)'"/1 -> dotprod44/1
  dotprod44/1 -> Mux/44
  "IW{1,1}(45,:)'"/1 -> dotprod45/1
  dotprod45/1 -> Mux/45
  "IW{1,1}(46,:)'"/1 -> dotprod46/1
  dotprod46/1 -> Mux/46
  "IW{1,1}(47,:)'"/1 -> dotprod47/1
  dotprod47/1 -> Mux/47
  "IW{1,1}(48,:)'"/1 -> dotprod48/1
  dotprod48/1 -> Mux/48
  "IW{1,1}(49,:)'"/1 -> dotprod49/1
  dotprod49/1 -> Mux/49
  "IW{1,1}(50,:)'"/1 -> dotprod50/1
  dotprod50/1 -> Mux/50
  "IW{1,1}(51,:)'"/1 -> dotprod51/1
  dotprod51/1 -> Mux/51
  "IW{1,1}(52,:)'"/1 -> dotprod52/1
  dotprod52/1 -> Mux/52
  "IW{1,1}(53,:)'"/1 -> dotprod53/1
  dotprod53/1 -> Mux/53
  "IW{1,1}(54,:)'"/1 -> dotprod54/1
  dotprod54/1 -> Mux/54
  "IW{1,1}(55,:)'"/1 -> dotprod55/1
  dotprod55/1 -> Mux/55
  Mux/1 -> "iz{1,1}"/1

== system ackerman_ROS_neural_controller/Controlador/Feed-Forward Neural Network/Layer 2/Delays 1 ==
  "p{2}" : Inport  PortDimensions=55
      mask Display: e = 0.06;c1 = [120 230 180]/255;c2 = ([120 230 180]+0)/(256+128);c3 = ([120 230 180]+128)/(256+128);patch([0 1 1 0],[0 0 1 1],c1);patch([0 1 1 1-e 1-e 0+e],[0 0 1 1-e 0+e 0+e],c2);patch([0 0 1 1-e 0+e 0+e],[0 1 1 1-e 1-e 0+e],c3);plot([0 1 1 0 0],[0 0 1 1 0]);
  mux : Mux  Inputs=1
      mask Display: e = 0.06;c1 = [120 150 230]/255;c2 = ([120 150 230]+0)/383;c3 = ([120 150 230]+128)/383;patch([0 1 1 0],[0 0 1 1],c1);patch([0 1 1 1-e 1-e 0+e],[0 0 1 1-e 0+e 0+e],c2);patch([0 0 1 1-e 0+e 0+e],[0 1 1 1-e 1-e 0+e],c3);plot([0 1 1 0 0],[0 0 1 1 0]);disp('Mux')
  "pd{2,1}" : Outport
      mask Display: e = 0.06;c1 = [120 230 180]/255;c2 = ([120 230 180]+0)/(256+128);c3 = ([120 230 180]+128)/(256+128);patch([0 1 1 0],[0 0 1 1],c1);patch([0 1 1 1-e 1-e 0+e],[0 0 1 1-e 0+e 0+e],c2);patch([0 0 1 1-e 0+e 0+e],[0 1 1 1-e 1-e 0+e],c3);plot([0 1 1 0 0],[0 0 1 1 0]);
  wires:
  "p{2}"/1 -> mux/1
  mux/1 -> "pd{2,1}"/1
